simulink model "ADU_Integration_Y2016_simulation"  (R2016b)
settings: Solver=FixedStepDiscrete  StartTime=240  StopTime=300  FixedStep=0.01  RelTol=1e-3  EnableMultiTasking=on
PostLoadFcn:
  | , if any(exist('dsrtsu_mdlpostloadfcn', 'file') == [2, 3, 6]), try dsrtsu_mdlpostloadfcn('Execute', bdroot); catch fprintf('Error in PostLoadFcn (dsrtsu_mdlpostloadfcn) for model "%s":\n %s\n', bdroot, lasterr); end, end,
InitFcn:
  | load 'data/chi2_dat';
  | load 'data/innerLine_struct';
  | load 'data/middleLine_struct';
  | load 'data/outerLine_struct';
  | load 'data/innerLine';
  | load 'data/middleLine';
  | load 'data/outerLine';
  | load 'data/landmarks_patac_schimmel_ccw';
  | load 'data/patac_navi_array';
  | load 'data/sensor';
  | load 'data/map_struct';
  | addpath map_src
  | Integration_Parameter;
  | load 'TestData_001';
values from neighbouring files (symbols this model uses):
  TestData_001 =     [TestData_001.mat]
undefined symbols (not defined in the file or in its folder): a, chi2_dat, innerLine, landmarks_patac_schimmel_ccw, middleLine, outerLine, patac_navi_array, StartNum
libraries: simulink x36, rtican x1
(part 6 of 20)

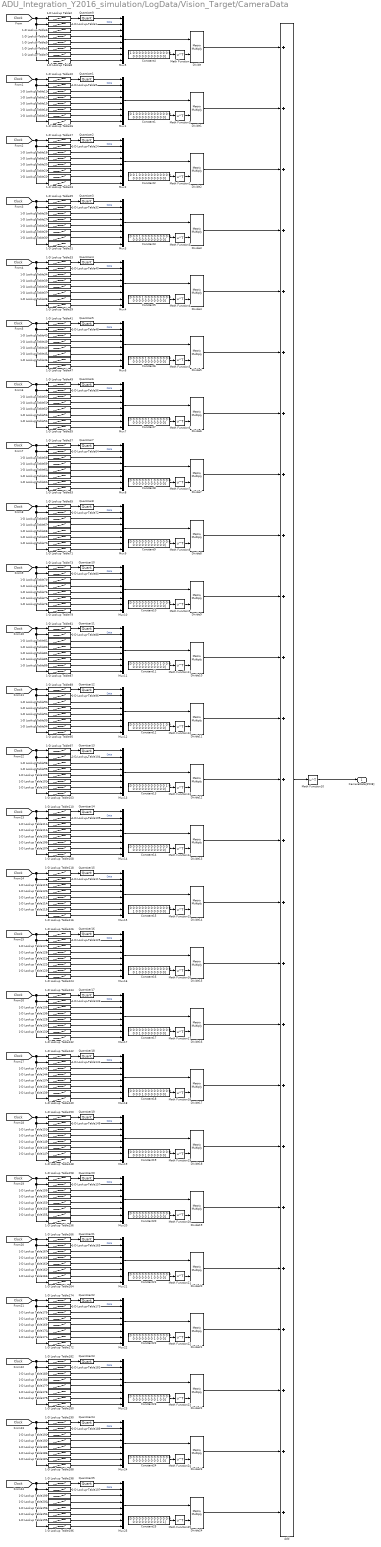
== system ADU_Integration_Y2016_simulation/LogData/Vision_Target/CameraData ==
  1-D Lookup Table1 : Lookup_n-D  NumberOfTableDimensions=1  BreakpointsForDimension1=TestData_001.X.Data  Table=TestData_001.Y(463+8*0).Data  RndMeth=Simplest  InputSameDT=on
  1-D Lookup Table10 : Lookup_n-D  NumberOfTableDimensions=1  BreakpointsForDimension1=TestData_001.X.Data  Table=TestData_001.Y(462+8*1).Data  RndMeth=Simplest  InputSameDT=on
  1-D Lookup Table100 : Lookup_n-D  NumberOfTableDimensions=1  BreakpointsForDimension1=TestData_001.X.Data  Table=TestData_001.Y(466+8*12).Data  RndMeth=Simplest  InputSameDT=on
  1-D Lookup Table101 : Lookup_n-D  NumberOfTableDimensions=1  BreakpointsForDimension1=TestData_001.X.Data  Table=TestData_001.Y(467+8*12).Data  RndMeth=Simplest  InputSameDT=on
  1-D Lookup Table102 : Lookup_n-D  NumberOfTableDimensions=1  BreakpointsForDimension1=TestData_001.X.Data  Table=TestData_001.Y(468+8*12).Data  RndMeth=Simplest  InputSameDT=on
  1-D Lookup Table103 : Lookup_n-D  NumberOfTableDimensions=1  BreakpointsForDimension1=TestData_001.X.Data  Table=TestData_001.Y(469+8*12).Data  RndMeth=Simplest  InputSameDT=on
  1-D Lookup Table104 : Lookup_n-D  NumberOfTableDimensions=1  BreakpointsForDimension1=TestData_001.X.Data  Table=TestData_001.Y(463+8*12).Data  RndMeth=Simplest  InputSameDT=on
  1-D Lookup Table105 : Lookup_n-D  NumberOfTableDimensions=1  BreakpointsForDimension1=TestData_001.X.Data  Table=TestData_001.Y(466+8*13).Data  RndMeth=Simplest  InputSameDT=on
  1-D Lookup Table106 : Lookup_n-D  NumberOfTableDimensions=1  BreakpointsForDimension1=TestData_001.X.Data  Table=TestData_001.Y(467+8*13).Data  RndMeth=Simplest  InputSameDT=on
  1-D Lookup Table107 : Lookup_n-D  NumberOfTableDimensions=1  BreakpointsForDimension1=TestData_001.X.Data  Table=TestData_001.Y(468+8*13).Data  RndMeth=Simplest  InputSameDT=on
  1-D Lookup Table108 : Lookup_n-D  NumberOfTableDimensions=1  BreakpointsForDimension1=TestData_001.X.Data  Table=TestData_001.Y(469+8*13).Data  RndMeth=Simplest  InputSameDT=on
  1-D Lookup Table109 : Lookup_n-D  NumberOfTableDimensions=1  BreakpointsForDimension1=TestData_001.X.Data  Table=TestData_001.Y(463+8*13).Data  RndMeth=Simplest  InputSameDT=on
  1-D Lookup Table11 : Lookup_n-D  NumberOfTableDimensions=1  BreakpointsForDimension1=TestData_001.X.Data  Table=TestData_001.Y(464+8*1).Data  RndMeth=Simplest  InputSameDT=on
  1-D Lookup Table110 : Lookup_n-D  NumberOfTableDimensions=1  BreakpointsForDimension1=TestData_001.X.Data  Table=TestData_001.Y(462+8*13).Data  RndMeth=Simplest  InputSameDT=on
  1-D Lookup Table111 : Lookup_n-D  NumberOfTableDimensions=1  BreakpointsForDimension1=TestData_001.X.Data  Table=TestData_001.Y(464+8*13).Data  RndMeth=Simplest  InputSameDT=on
  1-D Lookup Table112 : Lookup_n-D  NumberOfTableDimensions=1  BreakpointsForDimension1=TestData_001.X.Data  Table=TestData_001.Y(465+8*13).Data  RndMeth=Simplest  InputSameDT=on
  1-D Lookup Table113 : Lookup_n-D  NumberOfTableDimensions=1  BreakpointsForDimension1=TestData_001.X.Data  Table=TestData_001.Y(466+8*14).Data  RndMeth=Simplest  InputSameDT=on
  1-D Lookup Table114 : Lookup_n-D  NumberOfTableDimensions=1  BreakpointsForDimension1=TestData_001.X.Data  Table=TestData_001.Y(467+8*14).Data  RndMeth=Simplest  InputSameDT=on
  1-D Lookup Table115 : Lookup_n-D  NumberOfTableDimensions=1  BreakpointsForDimension1=TestData_001.X.Data  Table=TestData_001.Y(468+8*14).Data  RndMeth=Simplest  InputSameDT=on
  1-D Lookup Table116 : Lookup_n-D  NumberOfTableDimensions=1  BreakpointsForDimension1=TestData_001.X.Data  Table=TestData_001.Y(469+8*14).Data  RndMeth=Simplest  InputSameDT=on
  1-D Lookup Table117 : Lookup_n-D  NumberOfTableDimensions=1  BreakpointsForDimension1=TestData_001.X.Data  Table=TestData_001.Y(463+8*14).Data  RndMeth=Simplest  InputSameDT=on
  1-D Lookup Table118 : Lookup_n-D  NumberOfTableDimensions=1  BreakpointsForDimension1=TestData_001.X.Data  Table=TestData_001.Y(462+8*14).Data  RndMeth=Simplest  InputSameDT=on
  1-D Lookup Table119 : Lookup_n-D  NumberOfTableDimensions=1  BreakpointsForDimension1=TestData_001.X.Data  Table=TestData_001.Y(464+8*14).Data  RndMeth=Simplest  InputSameDT=on
  1-D Lookup Table12 : Lookup_n-D  NumberOfTableDimensions=1  BreakpointsForDimension1=TestData_001.X.Data  Table=TestData_001.Y(465+8*1).Data  RndMeth=Simplest  InputSameDT=on
  1-D Lookup Table120 : Lookup_n-D  NumberOfTableDimensions=1  BreakpointsForDimension1=TestData_001.X.Data  Table=TestData_001.Y(465+8*14).Data  RndMeth=Simplest  InputSameDT=on
  1-D Lookup Table121 : Lookup_n-D  NumberOfTableDimensions=1  BreakpointsForDimension1=TestData_001.X.Data  Table=TestData_001.Y(466+8*15).Data  RndMeth=Simplest  InputSameDT=on
  1-D Lookup Table122 : Lookup_n-D  NumberOfTableDimensions=1  BreakpointsForDimension1=TestData_001.X.Data  Table=TestData_001.Y(467+8*15).Data  RndMeth=Simplest  InputSameDT=on
  1-D Lookup Table123 : Lookup_n-D  NumberOfTableDimensions=1  BreakpointsForDimension1=TestData_001.X.Data  Table=TestData_001.Y(468+8*15).Data  RndMeth=Simplest  InputSameDT=on
  1-D Lookup Table124 : Lookup_n-D  NumberOfTableDimensions=1  BreakpointsForDimension1=TestData_001.X.Data  Table=TestData_001.Y(469+8*15).Data  RndMeth=Simplest  InputSameDT=on
  1-D Lookup Table125 : Lookup_n-D  NumberOfTableDimensions=1  BreakpointsForDimension1=TestData_001.X.Data  Table=TestData_001.Y(463+8*15).Data  RndMeth=Simplest  InputSameDT=on
  1-D Lookup Table126 : Lookup_n-D  NumberOfTableDimensions=1  BreakpointsForDimension1=TestData_001.X.Data  Table=TestData_001.Y(462+8*15).Data  RndMeth=Simplest  InputSameDT=on
  1-D Lookup Table127 : Lookup_n-D  NumberOfTableDimensions=1  BreakpointsForDimension1=TestData_001.X.Data  Table=TestData_001.Y(464+8*15).Data  RndMeth=Simplest  InputSameDT=on
  1-D Lookup Table128 : Lookup_n-D  NumberOfTableDimensions=1  BreakpointsForDimension1=TestData_001.X.Data  Table=TestData_001.Y(465+8*15).Data  RndMeth=Simplest  InputSameDT=on
  1-D Lookup Table129 : Lookup_n-D  NumberOfTableDimensions=1  BreakpointsForDimension1=TestData_001.X.Data  Table=TestData_001.Y(466+8*16).Data  RndMeth=Simplest  InputSameDT=on
  1-D Lookup Table13 : Lookup_n-D  NumberOfTableDimensions=1  BreakpointsForDimension1=TestData_001.X.Data  Table=TestData_001.Y(466+8*1).Data  RndMeth=Simplest  InputSameDT=on
  1-D Lookup Table130 : Lookup_n-D  NumberOfTableDimensions=1  BreakpointsForDimension1=TestData_001.X.Data  Table=TestData_001.Y(467+8*16).Data  RndMeth=Simplest  InputSameDT=on
  1-D Lookup Table131 : Lookup_n-D  NumberOfTableDimensions=1  BreakpointsForDimension1=TestData_001.X.Data  Table=TestData_001.Y(468+8*16).Data  RndMeth=Simplest  InputSameDT=on
  1-D Lookup Table132 : Lookup_n-D  NumberOfTableDimensions=1  BreakpointsForDimension1=TestData_001.X.Data  Table=TestData_001.Y(469+8*16).Data  RndMeth=Simplest  InputSameDT=on
  1-D Lookup Table133 : Lookup_n-D  NumberOfTableDimensions=1  BreakpointsForDimension1=TestData_001.X.Data  Table=TestData_001.Y(463+8*16).Data  RndMeth=Simplest  InputSameDT=on
  1-D Lookup Table134 : Lookup_n-D  NumberOfTableDimensions=1  BreakpointsForDimension1=TestData_001.X.Data  Table=TestData_001.Y(462+8*16).Data  RndMeth=Simplest  InputSameDT=on
  1-D Lookup Table135 : Lookup_n-D  NumberOfTableDimensions=1  BreakpointsForDimension1=TestData_001.X.Data  Table=TestData_001.Y(464+8*16).Data  RndMeth=Simplest  InputSameDT=on
  1-D Lookup Table136 : Lookup_n-D  NumberOfTableDimensions=1  BreakpointsForDimension1=TestData_001.X.Data  Table=TestData_001.Y(465+8*16).Data  RndMeth=Simplest  InputSameDT=on
  1-D Lookup Table137 : Lookup_n-D  NumberOfTableDimensions=1  BreakpointsForDimension1=TestData_001.X.Data  Table=TestData_001.Y(466+8*17).Data  RndMeth=Simplest  InputSameDT=on
  1-D Lookup Table138 : Lookup_n-D  NumberOfTableDimensions=1  BreakpointsForDimension1=TestData_001.X.Data  Table=TestData_001.Y(467+8*17).Data  RndMeth=Simplest  InputSameDT=on
  1-D Lookup Table139 : Lookup_n-D  NumberOfTableDimensions=1  BreakpointsForDimension1=TestData_001.X.Data  Table=TestData_001.Y(468+8*17).Data  RndMeth=Simplest  InputSameDT=on
  1-D Lookup Table14 : Lookup_n-D  NumberOfTableDimensions=1  BreakpointsForDimension1=TestData_001.X.Data  Table=TestData_001.Y(467+8*1).Data  RndMeth=Simplest  InputSameDT=on
  1-D Lookup Table140 : Lookup_n-D  NumberOfTableDimensions=1  BreakpointsForDimension1=TestData_001.X.Data  Table=TestData_001.Y(469+8*17).Data  RndMeth=Simplest  InputSameDT=on
  1-D Lookup Table141 : Lookup_n-D  NumberOfTableDimensions=1  BreakpointsForDimension1=TestData_001.X.Data  Table=TestData_001.Y(463+8*17).Data  RndMeth=Simplest  InputSameDT=on
  1-D Lookup Table142 : Lookup_n-D  NumberOfTableDimensions=1  BreakpointsForDimension1=TestData_001.X.Data  Table=TestData_001.Y(462+8*17).Data  RndMeth=Simplest  InputSameDT=on
  1-D Lookup Table143 : Lookup_n-D  NumberOfTableDimensions=1  BreakpointsForDimension1=TestData_001.X.Data  Table=TestData_001.Y(464+8*17).Data  RndMeth=Simplest  InputSameDT=on
  1-D Lookup Table144 : Lookup_n-D  NumberOfTableDimensions=1  BreakpointsForDimension1=TestData_001.X.Data  Table=TestData_001.Y(465+8*17).Data  RndMeth=Simplest  InputSameDT=on
  1-D Lookup Table145 : Lookup_n-D  NumberOfTableDimensions=1  BreakpointsForDimension1=TestData_001.X.Data  Table=TestData_001.Y(466+8*18).Data  RndMeth=Simplest  InputSameDT=on
  1-D Lookup Table146 : Lookup_n-D  NumberOfTableDimensions=1  BreakpointsForDimension1=TestData_001.X.Data  Table=TestData_001.Y(467+8*18).Data  RndMeth=Simplest  InputSameDT=on
  1-D Lookup Table147 : Lookup_n-D  NumberOfTableDimensions=1  BreakpointsForDimension1=TestData_001.X.Data  Table=TestData_001.Y(468+8*18).Data  RndMeth=Simplest  InputSameDT=on
  1-D Lookup Table148 : Lookup_n-D  NumberOfTableDimensions=1  BreakpointsForDimension1=TestData_001.X.Data  Table=TestData_001.Y(469+8*18).Data  RndMeth=Simplest  InputSameDT=on
  1-D Lookup Table149 : Lookup_n-D  NumberOfTableDimensions=1  BreakpointsForDimension1=TestData_001.X.Data  Table=TestData_001.Y(463+8*18).Data  RndMeth=Simplest  InputSameDT=on
  1-D Lookup Table15 : Lookup_n-D  NumberOfTableDimensions=1  BreakpointsForDimension1=TestData_001.X.Data  Table=TestData_001.Y(468+8*1).Data  RndMeth=Simplest  InputSameDT=on
  1-D Lookup Table150 : Lookup_n-D  NumberOfTableDimensions=1  BreakpointsForDimension1=TestData_001.X.Data  Table=TestData_001.Y(462+8*18).Data  RndMeth=Simplest  InputSameDT=on
  1-D Lookup Table151 : Lookup_n-D  NumberOfTableDimensions=1  BreakpointsForDimension1=TestData_001.X.Data  Table=TestData_001.Y(464+8*18).Data  RndMeth=Simplest  InputSameDT=on
  1-D Lookup Table152 : Lookup_n-D  NumberOfTableDimensions=1  BreakpointsForDimension1=TestData_001.X.Data  Table=TestData_001.Y(465+8*18).Data  RndMeth=Simplest  InputSameDT=on
  1-D Lookup Table153 : Lookup_n-D  NumberOfTableDimensions=1  BreakpointsForDimension1=TestData_001.X.Data  Table=TestData_001.Y(466+8*19).Data  RndMeth=Simplest  InputSameDT=on
  1-D Lookup Table154 : Lookup_n-D  NumberOfTableDimensions=1  BreakpointsForDimension1=TestData_001.X.Data  Table=TestData_001.Y(467+8*19).Data  RndMeth=Simplest  InputSameDT=on
  1-D Lookup Table155 : Lookup_n-D  NumberOfTableDimensions=1  BreakpointsForDimension1=TestData_001.X.Data  Table=TestData_001.Y(468+8*19).Data  RndMeth=Simplest  InputSameDT=on
  1-D Lookup Table156 : Lookup_n-D  NumberOfTableDimensions=1  BreakpointsForDimension1=TestData_001.X.Data  Table=TestData_001.Y(469+8*19).Data  RndMeth=Simplest  InputSameDT=on
  1-D Lookup Table157 : Lookup_n-D  NumberOfTableDimensions=1  BreakpointsForDimension1=TestData_001.X.Data  Table=TestData_001.Y(463+8*19).Data  RndMeth=Simplest  InputSameDT=on
  1-D Lookup Table158 : Lookup_n-D  NumberOfTableDimensions=1  BreakpointsForDimension1=TestData_001.X.Data  Table=TestData_001.Y(462+8*19).Data  RndMeth=Simplest  InputSameDT=on
  1-D Lookup Table159 : Lookup_n-D  NumberOfTableDimensions=1  BreakpointsForDimension1=TestData_001.X.Data  Table=TestData_001.Y(464+8*19).Data  RndMeth=Simplest  InputSameDT=on
  1-D Lookup Table16 : Lookup_n-D  NumberOfTableDimensions=1  BreakpointsForDimension1=TestData_001.X.Data  Table=TestData_001.Y(469+8*1).Data  RndMeth=Simplest  InputSameDT=on
  1-D Lookup Table160 : Lookup_n-D  NumberOfTableDimensions=1  BreakpointsForDimension1=TestData_001.X.Data  Table=TestData_001.Y(465+8*19).Data  RndMeth=Simplest  InputSameDT=on
  1-D Lookup Table161 : Lookup_n-D  NumberOfTableDimensions=1  BreakpointsForDimension1=TestData_001.X.Data  Table=TestData_001.Y(466+8*20).Data  RndMeth=Simplest  InputSameDT=on
  1-D Lookup Table162 : Lookup_n-D  NumberOfTableDimensions=1  BreakpointsForDimension1=TestData_001.X.Data  Table=TestData_001.Y(467+8*20).Data  RndMeth=Simplest  InputSameDT=on
  1-D Lookup Table163 : Lookup_n-D  NumberOfTableDimensions=1  BreakpointsForDimension1=TestData_001.X.Data  Table=TestData_001.Y(468+8*20).Data  RndMeth=Simplest  InputSameDT=on
  1-D Lookup Table164 : Lookup_n-D  NumberOfTableDimensions=1  BreakpointsForDimension1=TestData_001.X.Data  Table=TestData_001.Y(469+8*20).Data  RndMeth=Simplest  InputSameDT=on
  1-D Lookup Table165 : Lookup_n-D  NumberOfTableDimensions=1  BreakpointsForDimension1=TestData_001.X.Data  Table=TestData_001.Y(463+8*20).Data  RndMeth=Simplest  InputSameDT=on
  1-D Lookup Table166 : Lookup_n-D  NumberOfTableDimensions=1  BreakpointsForDimension1=TestData_001.X.Data  Table=TestData_001.Y(462+8*20).Data  RndMeth=Simplest  InputSameDT=on
  1-D Lookup Table167 : Lookup_n-D  NumberOfTableDimensions=1  BreakpointsForDimension1=TestData_001.X.Data  Table=TestData_001.Y(464+8*20).Data  RndMeth=Simplest  InputSameDT=on
  1-D Lookup Table168 : Lookup_n-D  NumberOfTableDimensions=1  BreakpointsForDimension1=TestData_001.X.Data  Table=TestData_001.Y(465+8*20).Data  RndMeth=Simplest  InputSameDT=on
  1-D Lookup Table169 : Lookup_n-D  NumberOfTableDimensions=1  BreakpointsForDimension1=TestData_001.X.Data  Table=TestData_001.Y(466+8*21).Data  RndMeth=Simplest  InputSameDT=on
  1-D Lookup Table17 : Lookup_n-D  NumberOfTableDimensions=1  BreakpointsForDimension1=TestData_001.X.Data  Table=TestData_001.Y(462+8*2).Data  RndMeth=Simplest  InputSameDT=on
  1-D Lookup Table170 : Lookup_n-D  NumberOfTableDimensions=1  BreakpointsForDimension1=TestData_001.X.Data  Table=TestData_001.Y(467+8*21).Data  RndMeth=Simplest  InputSameDT=on
  1-D Lookup Table171 : Lookup_n-D  NumberOfTableDimensions=1  BreakpointsForDimension1=TestData_001.X.Data  Table=TestData_001.Y(468+8*21).Data  RndMeth=Simplest  InputSameDT=on
  1-D Lookup Table172 : Lookup_n-D  NumberOfTableDimensions=1  BreakpointsForDimension1=TestData_001.X.Data  Table=TestData_001.Y(469+8*21).Data  RndMeth=Simplest  InputSameDT=on
  1-D Lookup Table173 : Lookup_n-D  NumberOfTableDimensions=1  BreakpointsForDimension1=TestData_001.X.Data  Table=TestData_001.Y(463+8*21).Data  RndMeth=Simplest  InputSameDT=on
  1-D Lookup Table174 : Lookup_n-D  NumberOfTableDimensions=1  BreakpointsForDimension1=TestData_001.X.Data  Table=TestData_001.Y(462+8*21).Data  RndMeth=Simplest  InputSameDT=on
  1-D Lookup Table175 : Lookup_n-D  NumberOfTableDimensions=1  BreakpointsForDimension1=TestData_001.X.Data  Table=TestData_001.Y(464+8*21).Data  RndMeth=Simplest  InputSameDT=on
  1-D Lookup Table176 : Lookup_n-D  NumberOfTableDimensions=1  BreakpointsForDimension1=TestData_001.X.Data  Table=TestData_001.Y(465+8*21).Data  RndMeth=Simplest  InputSameDT=on
  1-D Lookup Table177 : Lookup_n-D  NumberOfTableDimensions=1  BreakpointsForDimension1=TestData_001.X.Data  Table=TestData_001.Y(466+8*22).Data  RndMeth=Simplest  InputSameDT=on
  1-D Lookup Table178 : Lookup_n-D  NumberOfTableDimensions=1  BreakpointsForDimension1=TestData_001.X.Data  Table=TestData_001.Y(467+8*22).Data  RndMeth=Simplest  InputSameDT=on
  1-D Lookup Table179 : Lookup_n-D  NumberOfTableDimensions=1  BreakpointsForDimension1=TestData_001.X.Data  Table=TestData_001.Y(468+8*22).Data  RndMeth=Simplest  InputSameDT=on
  1-D Lookup Table18 : Lookup_n-D  NumberOfTableDimensions=1  BreakpointsForDimension1=TestData_001.X.Data  Table=TestData_001.Y(464+8*2).Data  RndMeth=Simplest  InputSameDT=on
  1-D Lookup Table180 : Lookup_n-D  NumberOfTableDimensions=1  BreakpointsForDimension1=TestData_001.X.Data  Table=TestData_001.Y(469+8*22).Data  RndMeth=Simplest  InputSameDT=on
  1-D Lookup Table181 : Lookup_n-D  NumberOfTableDimensions=1  BreakpointsForDimension1=TestData_001.X.Data  Table=TestData_001.Y(463+8*22).Data  RndMeth=Simplest  InputSameDT=on
  1-D Lookup Table182 : Lookup_n-D  NumberOfTableDimensions=1  BreakpointsForDimension1=TestData_001.X.Data  Table=TestData_001.Y(462+8*22).Data  RndMeth=Simplest  InputSameDT=on
  1-D Lookup Table183 : Lookup_n-D  NumberOfTableDimensions=1  BreakpointsForDimension1=TestData_001.X.Data  Table=TestData_001.Y(464+8*22).Data  RndMeth=Simplest  InputSameDT=on
  1-D Lookup Table184 : Lookup_n-D  NumberOfTableDimensions=1  BreakpointsForDimension1=TestData_001.X.Data  Table=TestData_001.Y(465+8*22).Data  RndMeth=Simplest  InputSameDT=on
  1-D Lookup Table185 : Lookup_n-D  NumberOfTableDimensions=1  BreakpointsForDimension1=TestData_001.X.Data  Table=TestData_001.Y(466+8*23).Data  RndMeth=Simplest  InputSameDT=on
  1-D Lookup Table186 : Lookup_n-D  NumberOfTableDimensions=1  BreakpointsForDimension1=TestData_001.X.Data  Table=TestData_001.Y(467+8*23).Data  RndMeth=Simplest  InputSameDT=on
  1-D Lookup Table187 : Lookup_n-D  NumberOfTableDimensions=1  BreakpointsForDimension1=TestData_001.X.Data  Table=TestData_001.Y(468+8*23).Data  RndMeth=Simplest  InputSameDT=on
  1-D Lookup Table188 : Lookup_n-D  NumberOfTableDimensions=1  BreakpointsForDimension1=TestData_001.X.Data  Table=TestData_001.Y(469+8*23).Data  RndMeth=Simplest  InputSameDT=on
  1-D Lookup Table189 : Lookup_n-D  NumberOfTableDimensions=1  BreakpointsForDimension1=TestData_001.X.Data  Table=TestData_001.Y(463+8*23).Data  RndMeth=Simplest  InputSameDT=on
  1-D Lookup Table19 : Lookup_n-D  NumberOfTableDimensions=1  BreakpointsForDimension1=TestData_001.X.Data  Table=TestData_001.Y(465+8*2).Data  RndMeth=Simplest  InputSameDT=on
  1-D Lookup Table190 : Lookup_n-D  NumberOfTableDimensions=1  BreakpointsForDimension1=TestData_001.X.Data  Table=TestData_001.Y(462+8*23).Data  RndMeth=Simplest  InputSameDT=on
  1-D Lookup Table191 : Lookup_n-D  NumberOfTableDimensions=1  BreakpointsForDimension1=TestData_001.X.Data  Table=TestData_001.Y(464+8*23).Data  RndMeth=Simplest  InputSameDT=on
  1-D Lookup Table192 : Lookup_n-D  NumberOfTableDimensions=1  BreakpointsForDimension1=TestData_001.X.Data  Table=TestData_001.Y(465+8*23).Data  RndMeth=Simplest  InputSameDT=on
  1-D Lookup Table193 : Lookup_n-D  NumberOfTableDimensions=1  BreakpointsForDimension1=TestData_001.X.Data  Table=TestData_001.Y(466+8*24).Data  RndMeth=Simplest  InputSameDT=on
  1-D Lookup Table194 : Lookup_n-D  NumberOfTableDimensions=1  BreakpointsForDimension1=TestData_001.X.Data  Table=TestData_001.Y(467+8*24).Data  RndMeth=Simplest  InputSameDT=on
  1-D Lookup Table195 : Lookup_n-D  NumberOfTableDimensions=1  BreakpointsForDimension1=TestData_001.X.Data  Table=TestData_001.Y(468+8*24).Data  RndMeth=Simplest  InputSameDT=on
  1-D Lookup Table196 : Lookup_n-D  NumberOfTableDimensions=1  BreakpointsForDimension1=TestData_001.X.Data  Table=TestData_001.Y(469+8*24).Data  RndMeth=Simplest  InputSameDT=on
  1-D Lookup Table197 : Lookup_n-D  NumberOfTableDimensions=1  BreakpointsForDimension1=TestData_001.X.Data  Table=TestData_001.Y(463+8*24).Data  RndMeth=Simplest  InputSameDT=on
  1-D Lookup Table198 : Lookup_n-D  NumberOfTableDimensions=1  BreakpointsForDimension1=TestData_001.X.Data  Table=TestData_001.Y(462+8*24).Data  RndMeth=Simplest  InputSameDT=on
  1-D Lookup Table199 : Lookup_n-D  NumberOfTableDimensions=1  BreakpointsForDimension1=TestData_001.X.Data  Table=TestData_001.Y(464+8*24).Data  RndMeth=Simplest  InputSameDT=on
  1-D Lookup Table2 : Lookup_n-D  NumberOfTableDimensions=1  BreakpointsForDimension1=TestData_001.X.Data  Table=TestData_001.Y(462+8*0).Data  RndMeth=Simplest  InputSameDT=on
  1-D Lookup Table20 : Lookup_n-D  NumberOfTableDimensions=1  BreakpointsForDimension1=TestData_001.X.Data  Table=TestData_001.Y(466+8*2).Data  RndMeth=Simplest  InputSameDT=on
  1-D Lookup Table200 : Lookup_n-D  NumberOfTableDimensions=1  BreakpointsForDimension1=TestData_001.X.Data  Table=TestData_001.Y(465+8*24).Data  RndMeth=Simplest  InputSameDT=on
  1-D Lookup Table21 : Lookup_n-D  NumberOfTableDimensions=1  BreakpointsForDimension1=TestData_001.X.Data  Table=TestData_001.Y(467+8*2).Data  RndMeth=Simplest  InputSameDT=on
  1-D Lookup Table22 : Lookup_n-D  NumberOfTableDimensions=1  BreakpointsForDimension1=TestData_001.X.Data  Table=TestData_001.Y(468+8*2).Data  RndMeth=Simplest  InputSameDT=on
  1-D Lookup Table23 : Lookup_n-D  NumberOfTableDimensions=1  BreakpointsForDimension1=TestData_001.X.Data  Table=TestData_001.Y(469+8*2).Data  RndMeth=Simplest  InputSameDT=on
  1-D Lookup Table24 : Lookup_n-D  NumberOfTableDimensions=1  BreakpointsForDimension1=TestData_001.X.Data  Table=TestData_001.Y(463+8*2).Data  RndMeth=Simplest  InputSameDT=on
  1-D Lookup Table25 : Lookup_n-D  NumberOfTableDimensions=1  BreakpointsForDimension1=TestData_001.X.Data  Table=TestData_001.Y(462+8*3).Data  RndMeth=Simplest  InputSameDT=on
  1-D Lookup Table26 : Lookup_n-D  NumberOfTableDimensions=1  BreakpointsForDimension1=TestData_001.X.Data  Table=TestData_001.Y(464+8*3).Data  RndMeth=Simplest  InputSameDT=on
  1-D Lookup Table27 : Lookup_n-D  NumberOfTableDimensions=1  BreakpointsForDimension1=TestData_001.X.Data  Table=TestData_001.Y(465+8*3).Data  RndMeth=Simplest  InputSameDT=on
  1-D Lookup Table28 : Lookup_n-D  NumberOfTableDimensions=1  BreakpointsForDimension1=TestData_001.X.Data  Table=TestData_001.Y(466+8*3).Data  RndMeth=Simplest  InputSameDT=on
  1-D Lookup Table29 : Lookup_n-D  NumberOfTableDimensions=1  BreakpointsForDimension1=TestData_001.X.Data  Table=TestData_001.Y(467+8*3).Data  RndMeth=Simplest  InputSameDT=on
  1-D Lookup Table3 : Lookup_n-D  NumberOfTableDimensions=1  BreakpointsForDimension1=TestData_001.X.Data  Table=TestData_001.Y(464+8*0).Data  RndMeth=Simplest  InputSameDT=on
  1-D Lookup Table30 : Lookup_n-D  NumberOfTableDimensions=1  BreakpointsForDimension1=TestData_001.X.Data  Table=TestData_001.Y(468+8*3).Data  RndMeth=Simplest  InputSameDT=on
  1-D Lookup Table31 : Lookup_n-D  NumberOfTableDimensions=1  BreakpointsForDimension1=TestData_001.X.Data  Table=TestData_001.Y(469+8*3).Data  RndMeth=Simplest  InputSameDT=on
  1-D Lookup Table32 : Lookup_n-D  NumberOfTableDimensions=1  BreakpointsForDimension1=TestData_001.X.Data  Table=TestData_001.Y(463+8*3).Data  RndMeth=Simplest  InputSameDT=on
  1-D Lookup Table33 : Lookup_n-D  NumberOfTableDimensions=1  BreakpointsForDimension1=TestData_001.X.Data  Table=TestData_001.Y(462+8*4).Data  RndMeth=Simplest  InputSameDT=on
  1-D Lookup Table34 : Lookup_n-D  NumberOfTableDimensions=1  BreakpointsForDimension1=TestData_001.X.Data  Table=TestData_001.Y(464+8*4).Data  RndMeth=Simplest  InputSameDT=on
  1-D Lookup Table35 : Lookup_n-D  NumberOfTableDimensions=1  BreakpointsForDimension1=TestData_001.X.Data  Table=TestData_001.Y(465+8*4).Data  RndMeth=Simplest  InputSameDT=on
  1-D Lookup Table36 : Lookup_n-D  NumberOfTableDimensions=1  BreakpointsForDimension1=TestData_001.X.Data  Table=TestData_001.Y(466+8*4).Data  RndMeth=Simplest  InputSameDT=on
  1-D Lookup Table37 : Lookup_n-D  NumberOfTableDimensions=1  BreakpointsForDimension1=TestData_001.X.Data  Table=TestData_001.Y(467+8*4).Data  RndMeth=Simplest  InputSameDT=on
  1-D Lookup Table38 : Lookup_n-D  NumberOfTableDimensions=1  BreakpointsForDimension1=TestData_001.X.Data  Table=TestData_001.Y(468+8*4).Data  RndMeth=Simplest  InputSameDT=on
  1-D Lookup Table39 : Lookup_n-D  NumberOfTableDimensions=1  BreakpointsForDimension1=TestData_001.X.Data  Table=TestData_001.Y(469+8*4).Data  RndMeth=Simplest  InputSameDT=on
  1-D Lookup Table4 : Lookup_n-D  NumberOfTableDimensions=1  BreakpointsForDimension1=TestData_001.X.Data  Table=TestData_001.Y(465+8*0).Data  RndMeth=Simplest  InputSameDT=on
  1-D Lookup Table40 : Lookup_n-D  NumberOfTableDimensions=1  BreakpointsForDimension1=TestData_001.X.Data  Table=TestData_001.Y(463+8*4).Data  RndMeth=Simplest  InputSameDT=on
  1-D Lookup Table41 : Lookup_n-D  NumberOfTableDimensions=1  BreakpointsForDimension1=TestData_001.X.Data  Table=TestData_001.Y(462+8*5).Data  RndMeth=Simplest  InputSameDT=on
  1-D Lookup Table42 : Lookup_n-D  NumberOfTableDimensions=1  BreakpointsForDimension1=TestData_001.X.Data  Table=TestData_001.Y(464+8*5).Data  RndMeth=Simplest  InputSameDT=on
  1-D Lookup Table43 : Lookup_n-D  NumberOfTableDimensions=1  BreakpointsForDimension1=TestData_001.X.Data  Table=TestData_001.Y(465+8*5).Data  RndMeth=Simplest  InputSameDT=on
  1-D Lookup Table44 : Lookup_n-D  NumberOfTableDimensions=1  BreakpointsForDimension1=TestData_001.X.Data  Table=TestData_001.Y(466+8*5).Data  RndMeth=Simplest  InputSameDT=on
  1-D Lookup Table45 : Lookup_n-D  NumberOfTableDimensions=1  BreakpointsForDimension1=TestData_001.X.Data  Table=TestData_001.Y(467+8*5).Data  RndMeth=Simplest  InputSameDT=on
  1-D Lookup Table46 : Lookup_n-D  NumberOfTableDimensions=1  BreakpointsForDimension1=TestData_001.X.Data  Table=TestData_001.Y(468+8*5).Data  RndMeth=Simplest  InputSameDT=on
  1-D Lookup Table47 : Lookup_n-D  NumberOfTableDimensions=1  BreakpointsForDimension1=TestData_001.X.Data  Table=TestData_001.Y(469+8*5).Data  RndMeth=Simplest  InputSameDT=on
  1-D Lookup Table48 : Lookup_n-D  NumberOfTableDimensions=1  BreakpointsForDimension1=TestData_001.X.Data  Table=TestData_001.Y(463+8*5).Data  RndMeth=Simplest  InputSameDT=on
  1-D Lookup Table49 : Lookup_n-D  NumberOfTableDimensions=1  BreakpointsForDimension1=TestData_001.X.Data  Table=TestData_001.Y(462+8*6).Data  RndMeth=Simplest  InputSameDT=on
  1-D Lookup Table5 : Lookup_n-D  NumberOfTableDimensions=1  BreakpointsForDimension1=TestData_001.X.Data  Table=TestData_001.Y(466+8*0).Data  RndMeth=Simplest  InputSameDT=on
  1-D Lookup Table50 : Lookup_n-D  NumberOfTableDimensions=1  BreakpointsForDimension1=TestData_001.X.Data  Table=TestData_001.Y(464+8*6).Data  RndMeth=Simplest  InputSameDT=on
  1-D Lookup Table51 : Lookup_n-D  NumberOfTableDimensions=1  BreakpointsForDimension1=TestData_001.X.Data  Table=TestData_001.Y(465+8*6).Data  RndMeth=Simplest  InputSameDT=on
  1-D Lookup Table52 : Lookup_n-D  NumberOfTableDimensions=1  BreakpointsForDimension1=TestData_001.X.Data  Table=TestData_001.Y(466+8*6).Data  RndMeth=Simplest  InputSameDT=on
  1-D Lookup Table53 : Lookup_n-D  NumberOfTableDimensions=1  BreakpointsForDimension1=TestData_001.X.Data  Table=TestData_001.Y(467+8*6).Data  RndMeth=Simplest  InputSameDT=on
  1-D Lookup Table54 : Lookup_n-D  NumberOfTableDimensions=1  BreakpointsForDimension1=TestData_001.X.Data  Table=TestData_001.Y(468+8*6).Data  RndMeth=Simplest  InputSameDT=on
  1-D Lookup Table55 : Lookup_n-D  NumberOfTableDimensions=1  BreakpointsForDimension1=TestData_001.X.Data  Table=TestData_001.Y(469+8*6).Data  RndMeth=Simplest  InputSameDT=on
  1-D Lookup Table56 : Lookup_n-D  NumberOfTableDimensions=1  BreakpointsForDimension1=TestData_001.X.Data  Table=TestData_001.Y(463+8*6).Data  RndMeth=Simplest  InputSameDT=on
  1-D Lookup Table57 : Lookup_n-D  NumberOfTableDimensions=1  BreakpointsForDimension1=TestData_001.X.Data  Table=TestData_001.Y(462+8*7).Data  RndMeth=Simplest  InputSameDT=on
  1-D Lookup Table58 : Lookup_n-D  NumberOfTableDimensions=1  BreakpointsForDimension1=TestData_001.X.Data  Table=TestData_001.Y(464+8*7).Data  RndMeth=Simplest  InputSameDT=on
  1-D Lookup Table59 : Lookup_n-D  NumberOfTableDimensions=1  BreakpointsForDimension1=TestData_001.X.Data  Table=TestData_001.Y(465+8*7).Data  RndMeth=Simplest  InputSameDT=on
  1-D Lookup Table6 : Lookup_n-D  NumberOfTableDimensions=1  BreakpointsForDimension1=TestData_001.X.Data  Table=TestData_001.Y(467+8*0).Data  RndMeth=Simplest  InputSameDT=on
  1-D Lookup Table60 : Lookup_n-D  NumberOfTableDimensions=1  BreakpointsForDimension1=TestData_001.X.Data  Table=TestData_001.Y(466+8*7).Data  RndMeth=Simplest  InputSameDT=on
  1-D Lookup Table61 : Lookup_n-D  NumberOfTableDimensions=1  BreakpointsForDimension1=TestData_001.X.Data  Table=TestData_001.Y(467+8*7).Data  RndMeth=Simplest  InputSameDT=on
  1-D Lookup Table62 : Lookup_n-D  NumberOfTableDimensions=1  BreakpointsForDimension1=TestData_001.X.Data  Table=TestData_001.Y(468+8*7).Data  RndMeth=Simplest  InputSameDT=on
  1-D Lookup Table63 : Lookup_n-D  NumberOfTableDimensions=1  BreakpointsForDimension1=TestData_001.X.Data  Table=TestData_001.Y(469+8*7).Data  RndMeth=Simplest  InputSameDT=on
  1-D Lookup Table64 : Lookup_n-D  NumberOfTableDimensions=1  BreakpointsForDimension1=TestData_001.X.Data  Table=TestData_001.Y(463+8*7).Data  RndMeth=Simplest  InputSameDT=on
  1-D Lookup Table65 : Lookup_n-D  NumberOfTableDimensions=1  BreakpointsForDimension1=TestData_001.X.Data  Table=TestData_001.Y(462+8*8).Data  RndMeth=Simplest  InputSameDT=on
  1-D Lookup Table66 : Lookup_n-D  NumberOfTableDimensions=1  BreakpointsForDimension1=TestData_001.X.Data  Table=TestData_001.Y(464+8*8).Data  RndMeth=Simplest  InputSameDT=on
  1-D Lookup Table67 : Lookup_n-D  NumberOfTableDimensions=1  BreakpointsForDimension1=TestData_001.X.Data  Table=TestData_001.Y(465+8*8).Data  RndMeth=Simplest  InputSameDT=on
  1-D Lookup Table68 : Lookup_n-D  NumberOfTableDimensions=1  BreakpointsForDimension1=TestData_001.X.Data  Table=TestData_001.Y(466+8*8).Data  RndMeth=Simplest  InputSameDT=on
  1-D Lookup Table69 : Lookup_n-D  NumberOfTableDimensions=1  BreakpointsForDimension1=TestData_001.X.Data  Table=TestData_001.Y(467+8*8).Data  RndMeth=Simplest  InputSameDT=on
  1-D Lookup Table7 : Lookup_n-D  NumberOfTableDimensions=1  BreakpointsForDimension1=TestData_001.X.Data  Table=TestData_001.Y(468+8*0).Data  RndMeth=Simplest  InputSameDT=on
  1-D Lookup Table70 : Lookup_n-D  NumberOfTableDimensions=1  BreakpointsForDimension1=TestData_001.X.Data  Table=TestData_001.Y(468+8*8).Data  RndMeth=Simplest  InputSameDT=on
  1-D Lookup Table71 : Lookup_n-D  NumberOfTableDimensions=1  BreakpointsForDimension1=TestData_001.X.Data  Table=TestData_001.Y(469+8*8).Data  RndMeth=Simplest  InputSameDT=on
  1-D Lookup Table72 : Lookup_n-D  NumberOfTableDimensions=1  BreakpointsForDimension1=TestData_001.X.Data  Table=TestData_001.Y(463+8*8).Data  RndMeth=Simplest  InputSameDT=on
  1-D Lookup Table73 : Lookup_n-D  NumberOfTableDimensions=1  BreakpointsForDimension1=TestData_001.X.Data  Table=TestData_001.Y(462+8*9).Data  RndMeth=Simplest  InputSameDT=on
  1-D Lookup Table74 : Lookup_n-D  NumberOfTableDimensions=1  BreakpointsForDimension1=TestData_001.X.Data  Table=TestData_001.Y(464+8*9).Data  RndMeth=Simplest  InputSameDT=on
  1-D Lookup Table75 : Lookup_n-D  NumberOfTableDimensions=1  BreakpointsForDimension1=TestData_001.X.Data  Table=TestData_001.Y(465+8*9).Data  RndMeth=Simplest  InputSameDT=on
  1-D Lookup Table76 : Lookup_n-D  NumberOfTableDimensions=1  BreakpointsForDimension1=TestData_001.X.Data  Table=TestData_001.Y(466+8*9).Data  RndMeth=Simplest  InputSameDT=on
  1-D Lookup Table77 : Lookup_n-D  NumberOfTableDimensions=1  BreakpointsForDimension1=TestData_001.X.Data  Table=TestData_001.Y(467+8*9).Data  RndMeth=Simplest  InputSameDT=on
  1-D Lookup Table78 : Lookup_n-D  NumberOfTableDimensions=1  BreakpointsForDimension1=TestData_001.X.Data  Table=TestData_001.Y(468+8*9).Data  RndMeth=Simplest  InputSameDT=on
  1-D Lookup Table79 : Lookup_n-D  NumberOfTableDimensions=1  BreakpointsForDimension1=TestData_001.X.Data  Table=TestData_001.Y(469+8*9).Data  RndMeth=Simplest  InputSameDT=on
  1-D Lookup Table8 : Lookup_n-D  NumberOfTableDimensions=1  BreakpointsForDimension1=TestData_001.X.Data  Table=TestData_001.Y(469+8*0).Data  RndMeth=Simplest  InputSameDT=on
  1-D Lookup Table80 : Lookup_n-D  NumberOfTableDimensions=1  BreakpointsForDimension1=TestData_001.X.Data  Table=TestData_001.Y(463+8*9).Data  RndMeth=Simplest  InputSameDT=on
  1-D Lookup Table81 : Lookup_n-D  NumberOfTableDimensions=1  BreakpointsForDimension1=TestData_001.X.Data  Table=TestData_001.Y(462+8*10).Data  RndMeth=Simplest  InputSameDT=on
  1-D Lookup Table82 : Lookup_n-D  NumberOfTableDimensions=1  BreakpointsForDimension1=TestData_001.X.Data  Table=TestData_001.Y(464+8*10).Data  RndMeth=Simplest  InputSameDT=on
  1-D Lookup Table83 : Lookup_n-D  NumberOfTableDimensions=1  BreakpointsForDimension1=TestData_001.X.Data  Table=TestData_001.Y(465+8*10).Data  RndMeth=Simplest  InputSameDT=on
  1-D Lookup Table84 : Lookup_n-D  NumberOfTableDimensions=1  BreakpointsForDimension1=TestData_001.X.Data  Table=TestData_001.Y(466+8*10).Data  RndMeth=Simplest  InputSameDT=on
  1-D Lookup Table85 : Lookup_n-D  NumberOfTableDimensions=1  BreakpointsForDimension1=TestData_001.X.Data  Table=TestData_001.Y(467+8*10).Data  RndMeth=Simplest  InputSameDT=on
  1-D Lookup Table86 : Lookup_n-D  NumberOfTableDimensions=1  BreakpointsForDimension1=TestData_001.X.Data  Table=TestData_001.Y(468+8*10).Data  RndMeth=Simplest  InputSameDT=on
  1-D Lookup Table87 : Lookup_n-D  NumberOfTableDimensions=1  BreakpointsForDimension1=TestData_001.X.Data  Table=TestData_001.Y(469+8*10).Data  RndMeth=Simplest  InputSameDT=on
  1-D Lookup Table88 : Lookup_n-D  NumberOfTableDimensions=1  BreakpointsForDimension1=TestData_001.X.Data  Table=TestData_001.Y(463+8*10).Data  RndMeth=Simplest  InputSameDT=on
  1-D Lookup Table89 : Lookup_n-D  NumberOfTableDimensions=1  BreakpointsForDimension1=TestData_001.X.Data  Table=TestData_001.Y(462+8*11).Data  RndMeth=Simplest  InputSameDT=on
  1-D Lookup Table9 : Lookup_n-D  NumberOfTableDimensions=1  BreakpointsForDimension1=TestData_001.X.Data  Table=TestData_001.Y(463+8*1).Data  RndMeth=Simplest  InputSameDT=on
  1-D Lookup Table90 : Lookup_n-D  NumberOfTableDimensions=1  BreakpointsForDimension1=TestData_001.X.Data  Table=TestData_001.Y(464+8*11).Data  RndMeth=Simplest  InputSameDT=on
  1-D Lookup Table91 : Lookup_n-D  NumberOfTableDimensions=1  BreakpointsForDimension1=TestData_001.X.Data  Table=TestData_001.Y(465+8*11).Data  RndMeth=Simplest  InputSameDT=on
  1-D Lookup Table92 : Lookup_n-D  NumberOfTableDimensions=1  BreakpointsForDimension1=TestData_001.X.Data  Table=TestData_001.Y(466+8*11).Data  RndMeth=Simplest  InputSameDT=on
  1-D Lookup Table93 : Lookup_n-D  NumberOfTableDimensions=1  BreakpointsForDimension1=TestData_001.X.Data  Table=TestData_001.Y(467+8*11).Data  RndMeth=Simplest  InputSameDT=on
  1-D Lookup Table94 : Lookup_n-D  NumberOfTableDimensions=1  BreakpointsForDimension1=TestData_001.X.Data  Table=TestData_001.Y(468+8*11).Data  RndMeth=Simplest  InputSameDT=on
  1-D Lookup Table95 : Lookup_n-D  NumberOfTableDimensions=1  BreakpointsForDimension1=TestData_001.X.Data  Table=TestData_001.Y(469+8*11).Data  RndMeth=Simplest  InputSameDT=on
  1-D Lookup Table96 : Lookup_n-D  NumberOfTableDimensions=1  BreakpointsForDimension1=TestData_001.X.Data  Table=TestData_001.Y(463+8*11).Data  RndMeth=Simplest  InputSameDT=on
  1-D Lookup Table97 : Lookup_n-D  NumberOfTableDimensions=1  BreakpointsForDimension1=TestData_001.X.Data  Table=TestData_001.Y(462+8*12).Data  RndMeth=Simplest  InputSameDT=on
  1-D Lookup Table98 : Lookup_n-D  NumberOfTableDimensions=1  BreakpointsForDimension1=TestData_001.X.Data  Table=TestData_001.Y(464+8*12).Data  RndMeth=Simplest  InputSameDT=on
  1-D Lookup Table99 : Lookup_n-D  NumberOfTableDimensions=1  BreakpointsForDimension1=TestData_001.X.Data  Table=TestData_001.Y(465+8*12).Data  RndMeth=Simplest  InputSameDT=on
  Add : Sum  Inputs=+++++++++++++++++++++++++
  Constant1 : Constant  Value=[0 1 0 0 0 0 0 0 0 0 0 0 0 0 0 0 0 0 0 0 0 0 0 0 0]
  Constant10 : Constant  Value=[0 0 0 0 0 0 0 0 0 1 0 0 0 0 0 0 0 0 0 0 0 0 0 0 0]
  Constant11 : Constant  Value=[0 0 0 0 0 0 0 0 0 0 1 0 0 0 0 0 0 0 0 0 0 0 0 0 0]
  Constant12 : Constant  Value=[0 0 0 0 0 0 0 0 0 0 0 1 0 0 0 0 0 0 0 0 0 0 0 0 0]
  Constant13 : Constant  Value=[0 0 0 0 0 0 0 0 0 0 0 0 1 0 0 0 0 0 0 0 0 0 0 0 0]
  Constant14 : Constant  Value=[0 0 0 0 0 0 0 0 0 0 0 0 0 1 0 0 0 0 0 0 0 0 0 0 0]
  Constant15 : Constant  Value=[0 0 0 0 0 0 0 0 0 0 0 0 0 0 1 0 0 0 0 0 0 0 0 0 0]
  Constant16 : Constant  Value=[0 0 0 0 0 0 0 0 0 0 0 0 0 0 0 1 0 0 0 0 0 0 0 0 0]
  Constant17 : Constant  Value=[0 0 0 0 0 0 0 0 0 0 0 0 0 0 0 0 1 0 0 0 0 0 0 0 0]
  Constant18 : Constant  Value=[0 0 0 0 0 0 0 0 0 0 0 0 0 0 0 0 0 1 0 0 0 0 0 0 0]
  Constant19 : Constant  Value=[0 0 0 0 0 0 0 0 0 0 0 0 0 0 0 0 0 0 1 0 0 0 0 0 0]
  Constant2 : Constant  Value=[0 0 1 0 0 0 0 0 0 0 0 0 0 0 0 0 0 0 0 0 0 0 0 0 0]
  Constant20 : Constant  Value=[0 0 0 0 0 0 0 0 0 0 0 0 0 0 0 0 0 0 0 1 0 0 0 0 0]
  Constant21 : Constant  Value=[0 0 0 0 0 0 0 0 0 0 0 0 0 0 0 0 0 0 0 0 1 0 0 0 0]
  Constant22 : Constant  Value=[0 0 0 0 0 0 0 0 0 0 0 0 0 0 0 0 0 0 0 0 0 1 0 0 0]
  Constant23 : Constant  Value=[0 0 0 0 0 0 0 0 0 0 0 0 0 0 0 0 0 0 0 0 0 0 1 0 0]
  Constant24 : Constant  Value=[0 0 0 0 0 0 0 0 0 0 0 0 0 0 0 0 0 0 0 0 0 0 0 1 0]
  Constant25 : Constant  Value=[0 0 0 0 0 0 0 0 0 0 0 0 0 0 0 0 0 0 0 0 0 0 0 0 1]
  Constant3 : Constant  Value=[0 0 0 1 0 0 0 0 0 0 0 0 0 0 0 0 0 0 0 0 0 0 0 0 0]
  Constant4 : Constant  Value=[1 0 0 0 0 0 0 0 0 0 0 0 0 0 0 0 0 0 0 0 0 0 0 0 0]
  Constant5 : Constant  Value=[0 0 0 0 1 0 0 0 0 0 0 0 0 0 0 0 0 0 0 0 0 0 0 0 0]
  Constant6 : Constant  Value=[0 0 0 0 0 1 0 0 0 0 0 0 0 0 0 0 0 0 0 0 0 0 0 0 0]
  Constant7 : Constant  Value=[0 0 0 0 0 0 1 0 0 0 0 0 0 0 0 0 0 0 0 0 0 0 0 0 0]
  Constant8 : Constant  Value=[0 0 0 0 0 0 0 1 0 0 0 0 0 0 0 0 0 0 0 0 0 0 0 0 0]
  Constant9 : Constant  Value=[0 0 0 0 0 0 0 0 1 0 0 0 0 0 0 0 0 0 0 0 0 0 0 0 0]
  Divide{,1..24} (25 alike) : Product  Inputs=**  Multiplication=Matrix(*)
  Math Function{,1..25} (26 alike) : Math  Operator=transpose  SaturateOnIntegerOverflow=on
  Mux{1..25} (25 alike) : Mux  Inputs=8
  Quantizer{1..25} (25 alike) : Quantizer  QuantizationInterval=1
  CameraData[25X8] : Outport
  wires:
  Mux5/1 -> Divide/1
  Constant4/1 -> Math Function/1
  Math Function/1 -> Divide/2
  Divide/1 -> Add/1
  Quantizer9/1 -> Mux5/1
  1-D Lookup Table4/1 -> Mux5/4
  1-D Lookup Table3/1 -> Mux5/3
  Add/1 -> Math Function10/1
  Math Function10/1 -> CameraData[25X8]/1
  1-D Lookup Table2/1 -> Quantizer9/1
  1-D Lookup Table1/1 -> Mux5/2  "Data"
  1-D Lookup Table5/1 -> Mux5/5
  1-D Lookup Table6/1 -> Mux5/6
  1-D Lookup Table7/1 -> Mux5/7
  [Clock] -> 1-D Lookup Table3/1, 1-D Lookup Table4/1, 1-D Lookup Table6/1, 1-D Lookup Table8/1, 1-D Lookup Table7/1, 1-D Lookup Table5/1, 1-D Lookup Table1/1, 1-D Lookup Table2/1
  1-D Lookup Table8/1 -> Mux5/8
  Mux1/1 -> Divide1/1
  Constant1/1 -> Math Function1/1
  Math Function1/1 -> Divide1/2
  Divide1/1 -> Add/2
  Quantizer1/1 -> Mux1/1
  1-D Lookup Table12/1 -> Mux1/4
  1-D Lookup Table11/1 -> Mux1/3
  1-D Lookup Table10/1 -> Quantizer1/1
  1-D Lookup Table9/1 -> Mux1/2  "Data"
  1-D Lookup Table13/1 -> Mux1/5
  1-D Lookup Table14/1 -> Mux1/6
  1-D Lookup Table15/1 -> Mux1/7
  [Clock] -> 1-D Lookup Table10/1, 1-D Lookup Table9/1, 1-D Lookup Table13/1, 1-D Lookup Table15/1, 1-D Lookup Table16/1, 1-D Lookup Table14/1, 1-D Lookup Table12/1, 1-D Lookup Table11/1
  1-D Lookup Table16/1 -> Mux1/8
  Mux2/1 -> Divide2/1
  Constant2/1 -> Math Function2/1
  Math Function2/1 -> Divide2/2
  Divide2/1 -> Add/3
  Quantizer2/1 -> Mux2/1
  1-D Lookup Table19/1 -> Mux2/4
  1-D Lookup Table18/1 -> Mux2/3
  1-D Lookup Table17/1 -> Quantizer2/1
  1-D Lookup Table24/1 -> Mux2/2  "Data"
  1-D Lookup Table20/1 -> Mux2/5
  1-D Lookup Table21/1 -> Mux2/6
  1-D Lookup Table22/1 -> Mux2/7
  [Clock] -> 1-D Lookup Table18/1, 1-D Lookup Table19/1, 1-D Lookup Table21/1, 1-D Lookup Table23/1, 1-D Lookup Table22/1, 1-D Lookup Table20/1, 1-D Lookup Table24/1, 1-D Lookup Table17/1
  1-D Lookup Table23/1 -> Mux2/8
  Mux3/1 -> Divide3/1
  Constant3/1 -> Math Function3/1
  Math Function3/1 -> Divide3/2
  Divide3/1 -> Add/4
  Quantizer3/1 -> Mux3/1
  1-D Lookup Table27/1 -> Mux3/4
  1-D Lookup Table26/1 -> Mux3/3
  1-D Lookup Table25/1 -> Quantizer3/1
  1-D Lookup Table32/1 -> Mux3/2  "Data"
  1-D Lookup Table28/1 -> Mux3/5
  1-D Lookup Table29/1 -> Mux3/6
  1-D Lookup Table30/1 -> Mux3/7
  [Clock] -> 1-D Lookup Table25/1, 1-D Lookup Table32/1, 1-D Lookup Table28/1, 1-D Lookup Table30/1, 1-D Lookup Table31/1, 1-D Lookup Table29/1, 1-D Lookup Table27/1, 1-D Lookup Table26/1
  1-D Lookup Table31/1 -> Mux3/8
  Mux4/1 -> Divide4/1
  Constant5/1 -> Math Function4/1
  Math Function4/1 -> Divide4/2
  Divide4/1 -> Add/5
  Quantizer4/1 -> Mux4/1
  1-D Lookup Table35/1 -> Mux4/4
  1-D Lookup Table34/1 -> Mux4/3
  1-D Lookup Table33/1 -> Quantizer4/1
  1-D Lookup Table40/1 -> Mux4/2  "Data"
  1-D Lookup Table36/1 -> Mux4/5
  1-D Lookup Table37/1 -> Mux4/6
  1-D Lookup Table38/1 -> Mux4/7
  [Clock] -> 1-D Lookup Table34/1, 1-D Lookup Table35/1, 1-D Lookup Table37/1, 1-D Lookup Table39/1, 1-D Lookup Table38/1, 1-D Lookup Table36/1, 1-D Lookup Table40/1, 1-D Lookup Table33/1
  1-D Lookup Table39/1 -> Mux4/8
  Mux6/1 -> Divide5/1
  Constant6/1 -> Math Function5/1
  Math Function5/1 -> Divide5/2
  Divide5/1 -> Add/6
  Quantizer5/1 -> Mux6/1
  1-D Lookup Table43/1 -> Mux6/4
  1-D Lookup Table42/1 -> Mux6/3
  1-D Lookup Table41/1 -> Quantizer5/1
  1-D Lookup Table48/1 -> Mux6/2  "Data"
  1-D Lookup Table44/1 -> Mux6/5
  1-D Lookup Table45/1 -> Mux6/6
  1-D Lookup Table46/1 -> Mux6/7
  [Clock] -> 1-D Lookup Table41/1, 1-D Lookup Table48/1, 1-D Lookup Table44/1, 1-D Lookup Table46/1, 1-D Lookup Table47/1, 1-D Lookup Table45/1, 1-D Lookup Table43/1, 1-D Lookup Table42/1
  1-D Lookup Table47/1 -> Mux6/8
  Mux7/1 -> Divide6/1
  Constant7/1 -> Math Function6/1
  Math Function6/1 -> Divide6/2
  Divide6/1 -> Add/7
  Quantizer6/1 -> Mux7/1
  1-D Lookup Table51/1 -> Mux7/4
  1-D Lookup Table50/1 -> Mux7/3
  1-D Lookup Table49/1 -> Quantizer6/1
  1-D Lookup Table56/1 -> Mux7/2  "Data"
  1-D Lookup Table52/1 -> Mux7/5
  1-D Lookup Table53/1 -> Mux7/6
  1-D Lookup Table54/1 -> Mux7/7
  [Clock] -> 1-D Lookup Table50/1, 1-D Lookup Table51/1, 1-D Lookup Table53/1, 1-D Lookup Table55/1, 1-D Lookup Table54/1, 1-D Lookup Table52/1, 1-D Lookup Table56/1, 1-D Lookup Table49/1
  1-D Lookup Table55/1 -> Mux7/8
  Mux8/1 -> Divide7/1
  Constant8/1 -> Math Function7/1
  Math Function7/1 -> Divide7/2
  Divide7/1 -> Add/8
  Quantizer7/1 -> Mux8/1
  1-D Lookup Table59/1 -> Mux8/4
  1-D Lookup Table58/1 -> Mux8/3
  1-D Lookup Table57/1 -> Quantizer7/1
  1-D Lookup Table64/1 -> Mux8/2  "Data"
  1-D Lookup Table60/1 -> Mux8/5
  1-D Lookup Table61/1 -> Mux8/6
  1-D Lookup Table62/1 -> Mux8/7
  [Clock] -> 1-D Lookup Table57/1, 1-D Lookup Table64/1, 1-D Lookup Table60/1, 1-D Lookup Table62/1, 1-D Lookup Table63/1, 1-D Lookup Table61/1, 1-D Lookup Table59/1, 1-D Lookup Table58/1
  1-D Lookup Table63/1 -> Mux8/8
  Mux9/1 -> Divide8/1
  Constant9/1 -> Math Function8/1
  Math Function8/1 -> Divide8/2
  Divide8/1 -> Add/9
  Quantizer8/1 -> Mux9/1
  1-D Lookup Table67/1 -> Mux9/4
  1-D Lookup Table66/1 -> Mux9/3
  1-D Lookup Table65/1 -> Quantizer8/1
  1-D Lookup Table72/1 -> Mux9/2  "Data"
  1-D Lookup Table68/1 -> Mux9/5
  1-D Lookup Table69/1 -> Mux9/6
  1-D Lookup Table70/1 -> Mux9/7
  [Clock] -> 1-D Lookup Table66/1, 1-D Lookup Table67/1, 1-D Lookup Table69/1, 1-D Lookup Table71/1, 1-D Lookup Table70/1, 1-D Lookup Table68/1, 1-D Lookup Table72/1, 1-D Lookup Table65/1
  1-D Lookup Table71/1 -> Mux9/8
  Mux10/1 -> Divide9/1
  Constant10/1 -> Math Function9/1
  Math Function9/1 -> Divide9/2
  Divide9/1 -> Add/10
  Quantizer10/1 -> Mux10/1
  1-D Lookup Table75/1 -> Mux10/4
  1-D Lookup Table74/1 -> Mux10/3
  1-D Lookup Table73/1 -> Quantizer10/1
  1-D Lookup Table80/1 -> Mux10/2  "Data"
  1-D Lookup Table76/1 -> Mux10/5
  1-D Lookup Table77/1 -> Mux10/6
  1-D Lookup Table78/1 -> Mux10/7
  [Clock] -> 1-D Lookup Table73/1, 1-D Lookup Table80/1, 1-D Lookup Table76/1, 1-D Lookup Table78/1, 1-D Lookup Table79/1, 1-D Lookup Table77/1, 1-D Lookup Table75/1, 1-D Lookup Table74/1
  1-D Lookup Table79/1 -> Mux10/8
  Mux11/1 -> Divide10/1
  Constant11/1 -> Math Function11/1
  Math Function11/1 -> Divide10/2
  Divide10/1 -> Add/11
  Quantizer11/1 -> Mux11/1
  1-D Lookup Table83/1 -> Mux11/4
  1-D Lookup Table82/1 -> Mux11/3
  1-D Lookup Table81/1 -> Quantizer11/1
  1-D Lookup Table88/1 -> Mux11/2  "Data"
  1-D Lookup Table84/1 -> Mux11/5
  1-D Lookup Table85/1 -> Mux11/6
  1-D Lookup Table86/1 -> Mux11/7
  [Clock] -> 1-D Lookup Table82/1, 1-D Lookup Table83/1, 1-D Lookup Table85/1, 1-D Lookup Table87/1, 1-D Lookup Table86/1, 1-D Lookup Table84/1, 1-D Lookup Table88/1, 1-D Lookup Table81/1
  1-D Lookup Table87/1 -> Mux11/8
  Mux12/1 -> Divide11/1
  Constant12/1 -> Math Function12/1
  Math Function12/1 -> Divide11/2
  Divide11/1 -> Add/12
  Quantizer12/1 -> Mux12/1
  1-D Lookup Table91/1 -> Mux12/4
  1-D Lookup Table90/1 -> Mux12/3
  1-D Lookup Table89/1 -> Quantizer12/1
  1-D Lookup Table96/1 -> Mux12/2  "Data"
  1-D Lookup Table92/1 -> Mux12/5
  1-D Lookup Table93/1 -> Mux12/6
  1-D Lookup Table94/1 -> Mux12/7
  [Clock] -> 1-D Lookup Table89/1, 1-D Lookup Table96/1, 1-D Lookup Table92/1, 1-D Lookup Table94/1, 1-D Lookup Table95/1, 1-D Lookup Table93/1, 1-D Lookup Table91/1, 1-D Lookup Table90/1
  1-D Lookup Table95/1 -> Mux12/8
  Mux13/1 -> Divide12/1
  Constant13/1 -> Math Function13/1
  Math Function13/1 -> Divide12/2
  Divide12/1 -> Add/13
  Quantizer13/1 -> Mux13/1
  1-D Lookup Table99/1 -> Mux13/4
  1-D Lookup Table98/1 -> Mux13/3
  1-D Lookup Table97/1 -> Quantizer13/1
  1-D Lookup Table104/1 -> Mux13/2  "Data"
  1-D Lookup Table100/1 -> Mux13/5
  1-D Lookup Table101/1 -> Mux13/6
  1-D Lookup Table102/1 -> Mux13/7
  [Clock] -> 1-D Lookup Table98/1, 1-D Lookup Table99/1, 1-D Lookup Table101/1, 1-D Lookup Table103/1, 1-D Lookup Table102/1, 1-D Lookup Table100/1, 1-D Lookup Table104/1, 1-D Lookup Table97/1
  1-D Lookup Table103/1 -> Mux13/8
  Mux14/1 -> Divide13/1
  Constant14/1 -> Math Function14/1
  Math Function14/1 -> Divide13/2
  Divide13/1 -> Add/14
  Quantizer14/1 -> Mux14/1
  1-D Lookup Table112/1 -> Mux14/4
  1-D Lookup Table111/1 -> Mux14/3
  1-D Lookup Table110/1 -> Quantizer14/1
  1-D Lookup Table109/1 -> Mux14/2  "Data"
  1-D Lookup Table105/1 -> Mux14/5
  1-D Lookup Table106/1 -> Mux14/6
  1-D Lookup Table107/1 -> Mux14/7
  [Clock] -> 1-D Lookup Table110/1, 1-D Lookup Table109/1, 1-D Lookup Table105/1, 1-D Lookup Table107/1, 1-D Lookup Table108/1, 1-D Lookup Table106/1, 1-D Lookup Table112/1, 1-D Lookup Table111/1
  1-D Lookup Table108/1 -> Mux14/8
  Mux15/1 -> Divide14/1
  Constant15/1 -> Math Function15/1
  Math Function15/1 -> Divide14/2
  Divide14/1 -> Add/15
  Quantizer15/1 -> Mux15/1
  1-D Lookup Table120/1 -> Mux15/4
  1-D Lookup Table119/1 -> Mux15/3
  1-D Lookup Table118/1 -> Quantizer15/1
  1-D Lookup Table117/1 -> Mux15/2  "Data"
  1-D Lookup Table113/1 -> Mux15/5
  1-D Lookup Table114/1 -> Mux15/6
  1-D Lookup Table115/1 -> Mux15/7
  [Clock] -> 1-D Lookup Table119/1, 1-D Lookup Table120/1, 1-D Lookup Table114/1, 1-D Lookup Table116/1, 1-D Lookup Table115/1, 1-D Lookup Table113/1, 1-D Lookup Table117/1, 1-D Lookup Table118/1
  1-D Lookup Table116/1 -> Mux15/8
  Mux16/1 -> Divide15/1
  Constant16/1 -> Math Function16/1
  Math Function16/1 -> Divide15/2
  Divide15/1 -> Add/16
  Quantizer16/1 -> Mux16/1
  1-D Lookup Table128/1 -> Mux16/4
  1-D Lookup Table127/1 -> Mux16/3
  1-D Lookup Table126/1 -> Quantizer16/1
  1-D Lookup Table125/1 -> Mux16/2  "Data"
  1-D Lookup Table121/1 -> Mux16/5
  1-D Lookup Table122/1 -> Mux16/6
  1-D Lookup Table123/1 -> Mux16/7
  [Clock] -> 1-D Lookup Table126/1, 1-D Lookup Table125/1, 1-D Lookup Table121/1, 1-D Lookup Table123/1, 1-D Lookup Table124/1, 1-D Lookup Table122/1, 1-D Lookup Table128/1, 1-D Lookup Table127/1
  1-D Lookup Table124/1 -> Mux16/8
  Mux17/1 -> Divide16/1
  Constant17/1 -> Math Function17/1
  Math Function17/1 -> Divide16/2
  Divide16/1 -> Add/17
  Quantizer17/1 -> Mux17/1
  1-D Lookup Table136/1 -> Mux17/4
  1-D Lookup Table135/1 -> Mux17/3
  1-D Lookup Table134/1 -> Quantizer17/1
  1-D Lookup Table133/1 -> Mux17/2  "Data"
  1-D Lookup Table129/1 -> Mux17/5
  1-D Lookup Table130/1 -> Mux17/6
  1-D Lookup Table131/1 -> Mux17/7
  [Clock] -> 1-D Lookup Table135/1, 1-D Lookup Table136/1, 1-D Lookup Table130/1, 1-D Lookup Table132/1, 1-D Lookup Table131/1, 1-D Lookup Table129/1, 1-D Lookup Table133/1, 1-D Lookup Table134/1
  1-D Lookup Table132/1 -> Mux17/8
  Mux18/1 -> Divide17/1
  Constant18/1 -> Math Function18/1
  Math Function18/1 -> Divide17/2
  Divide17/1 -> Add/18
  Quantizer18/1 -> Mux18/1
  1-D Lookup Table144/1 -> Mux18/4
  1-D Lookup Table143/1 -> Mux18/3
  1-D Lookup Table142/1 -> Quantizer18/1
  1-D Lookup Table141/1 -> Mux18/2  "Data"
  1-D Lookup Table137/1 -> Mux18/5
  1-D Lookup Table138/1 -> Mux18/6
  1-D Lookup Table139/1 -> Mux18/7
  [Clock] -> 1-D Lookup Table142/1, 1-D Lookup Table141/1, 1-D Lookup Table137/1, 1-D Lookup Table139/1, 1-D Lookup Table140/1, 1-D Lookup Table138/1, 1-D Lookup Table144/1, 1-D Lookup Table143/1
  1-D Lookup Table140/1 -> Mux18/8
  Mux19/1 -> Divide18/1
  Constant19/1 -> Math Function19/1
  Math Function19/1 -> Divide18/2
  Divide18/1 -> Add/19
  Quantizer19/1 -> Mux19/1
  1-D Lookup Table152/1 -> Mux19/4
  1-D Lookup Table151/1 -> Mux19/3
  1-D Lookup Table150/1 -> Quantizer19/1
  1-D Lookup Table149/1 -> Mux19/2  "Data"
  1-D Lookup Table145/1 -> Mux19/5
  1-D Lookup Table146/1 -> Mux19/6
  1-D Lookup Table147/1 -> Mux19/7
  [Clock] -> 1-D Lookup Table151/1, 1-D Lookup Table152/1, 1-D Lookup Table146/1, 1-D Lookup Table148/1, 1-D Lookup Table147/1, 1-D Lookup Table145/1, 1-D Lookup Table149/1, 1-D Lookup Table150/1
  1-D Lookup Table148/1 -> Mux19/8
  Mux20/1 -> Divide19/1
  Constant20/1 -> Math Function20/1
  Math Function20/1 -> Divide19/2
  Divide19/1 -> Add/20
  Quantizer20/1 -> Mux20/1
  1-D Lookup Table160/1 -> Mux20/4
  1-D Lookup Table159/1 -> Mux20/3
  1-D Lookup Table158/1 -> Quantizer20/1
  1-D Lookup Table157/1 -> Mux20/2  "Data"
  1-D Lookup Table153/1 -> Mux20/5
  1-D Lookup Table154/1 -> Mux20/6
  1-D Lookup Table155/1 -> Mux20/7
  [Clock] -> 1-D Lookup Table158/1, 1-D Lookup Table157/1, 1-D Lookup Table153/1, 1-D Lookup Table155/1, 1-D Lookup Table156/1, 1-D Lookup Table154/1, 1-D Lookup Table160/1, 1-D Lookup Table159/1
  1-D Lookup Table156/1 -> Mux20/8
  Mux21/1 -> Divide20/1
  Constant21/1 -> Math Function21/1
  Math Function21/1 -> Divide20/2
  Divide20/1 -> Add/21
  Quantizer21/1 -> Mux21/1
  1-D Lookup Table168/1 -> Mux21/4
  1-D Lookup Table167/1 -> Mux21/3
  1-D Lookup Table166/1 -> Quantizer21/1
  1-D Lookup Table165/1 -> Mux21/2  "Data"
  1-D Lookup Table161/1 -> Mux21/5
  1-D Lookup Table162/1 -> Mux21/6
  1-D Lookup Table163/1 -> Mux21/7
  [Clock] -> 1-D Lookup Table167/1, 1-D Lookup Table168/1, 1-D Lookup Table162/1, 1-D Lookup Table164/1, 1-D Lookup Table163/1, 1-D Lookup Table161/1, 1-D Lookup Table165/1, 1-D Lookup Table166/1
  1-D Lookup Table164/1 -> Mux21/8
  Mux22/1 -> Divide21/1
  Constant22/1 -> Math Function22/1
  Math Function22/1 -> Divide21/2
  Divide21/1 -> Add/22
  Quantizer22/1 -> Mux22/1
  1-D Lookup Table176/1 -> Mux22/4
  1-D Lookup Table175/1 -> Mux22/3
  1-D Lookup Table174/1 -> Quantizer22/1
  1-D Lookup Table173/1 -> Mux22/2  "Data"
  1-D Lookup Table169/1 -> Mux22/5
  1-D Lookup Table170/1 -> Mux22/6
  1-D Lookup Table171/1 -> Mux22/7
  [Clock] -> 1-D Lookup Table174/1, 1-D Lookup Table173/1, 1-D Lookup Table169/1, 1-D Lookup Table171/1, 1-D Lookup Table172/1, 1-D Lookup Table170/1, 1-D Lookup Table176/1, 1-D Lookup Table175/1
  1-D Lookup Table172/1 -> Mux22/8
  Mux23/1 -> Divide22/1
  Constant23/1 -> Math Function23/1
  Math Function23/1 -> Divide22/2
  Divide22/1 -> Add/23
  Quantizer23/1 -> Mux23/1
  1-D Lookup Table184/1 -> Mux23/4
  1-D Lookup Table183/1 -> Mux23/3
  1-D Lookup Table182/1 -> Quantizer23/1
  1-D Lookup Table181/1 -> Mux23/2  "Data"
  1-D Lookup Table177/1 -> Mux23/5
  1-D Lookup Table178/1 -> Mux23/6
  1-D Lookup Table179/1 -> Mux23/7
  [Clock] -> 1-D Lookup Table183/1, 1-D Lookup Table184/1, 1-D Lookup Table178/1, 1-D Lookup Table180/1, 1-D Lookup Table179/1, 1-D Lookup Table177/1, 1-D Lookup Table181/1, 1-D Lookup Table182/1
  1-D Lookup Table180/1 -> Mux23/8
  Mux24/1 -> Divide23/1
  Constant24/1 -> Math Function24/1
  Math Function24/1 -> Divide23/2
  Divide23/1 -> Add/24
  Quantizer24/1 -> Mux24/1
  1-D Lookup Table192/1 -> Mux24/4
  1-D Lookup Table191/1 -> Mux24/3
  1-D Lookup Table190/1 -> Quantizer24/1
  1-D Lookup Table189/1 -> Mux24/2  "Data"
  1-D Lookup Table185/1 -> Mux24/5
  1-D Lookup Table186/1 -> Mux24/6
  1-D Lookup Table187/1 -> Mux24/7
  [Clock] -> 1-D Lookup Table190/1, 1-D Lookup Table189/1, 1-D Lookup Table185/1, 1-D Lookup Table187/1, 1-D Lookup Table188/1, 1-D Lookup Table186/1, 1-D Lookup Table192/1, 1-D Lookup Table191/1
  1-D Lookup Table188/1 -> Mux24/8
  Mux25/1 -> Divide24/1
  Constant25/1 -> Math Function25/1
  Math Function25/1 -> Divide24/2
  Divide24/1 -> Add/25
  Quantizer25/1 -> Mux25/1
  1-D Lookup Table200/1 -> Mux25/4
  1-D Lookup Table199/1 -> Mux25/3
  1-D Lookup Table198/1 -> Quantizer25/1
  1-D Lookup Table197/1 -> Mux25/2  "Data"
  1-D Lookup Table193/1 -> Mux25/5
  1-D Lookup Table194/1 -> Mux25/6
  1-D Lookup Table195/1 -> Mux25/7
  [Clock] -> 1-D Lookup Table199/1, 1-D Lookup Table200/1, 1-D Lookup Table194/1, 1-D Lookup Table196/1, 1-D Lookup Table195/1, 1-D Lookup Table193/1, 1-D Lookup Table197/1, 1-D Lookup Table198/1
  1-D Lookup Table196/1 -> Mux25/8
